simulink model "VSCMGs_trackingOrbital"  (R2019b)
settings: Solver=ode45  StartTime=0.0  StopTime=tf  FixedStep=0.01  MaxStep=0.1  RelTol=10^(-6)  EnableMultiTasking=on
InitFcn:
  | initialize
StopFcn:
  | plotting
values from neighbouring files (symbols this model uses):
  g10 = [1; 0; 0]    [initialize.m]
  g20 = [0; 1; 0]    [initialize.m]
  g30 = [0; 0; 1]    [initialize.m]
  gamma10 = 0    [initialize.m]
  gamma20 = 0    [initialize.m]
  gamma30 = 0    [initialize.m]
  h = cross(r0, v0)    [initialize.m]
  Isw = 0.1    [initialize.m]
  J = [87.252, 0, 0; 0, 85.07, 0; 0, 0, 113.565]    [initialize.m]
  K = 10^(1)*eye(3)    [initialize.m]
  mu = 10^(-20)    (= 1e-20)    [initialize.m]
  mugrav = G*(m1+m2)    (= 398583.224)    [initialize.m]
  om0 = [0; 0; 0]*(2*pi/60)    [initialize.m]
  Om0 = [500; 500; 500]*2*pi/60    [initialize.m]
  q0 = [0; 0; 0; 1]    [initialize.m]
  r0 = [8000; 0; 6000]    [initialize.m]
  s10 = [0; 1; 0]    [initialize.m]
  s20 = [1; 0; 0]    [initialize.m]
  s30 = [0; 1; 0]    [initialize.m]
  t10 = [0; 0; 1]    [initialize.m]
  t20 = [0; 0; -1]    [initialize.m]
  t30 = [-1; 0; 0]    [initialize.m]
  v0 = [0; 8.5; 0]    [initialize.m]
  Wg0 = 1    [initialize.m]
  Ws0 = 200    [initialize.m]
  Y = [0.03, 0, 0; 0, 0.13, 0; 0, 0, 0.04]    [initialize.m]
settings Model: Creator=bevilr  LastModifiedBy=bevilr
settings DataIOCC: ReturnWorkspaceOutputs=off
settings OptimizationCC: LifeSpan=inf
settings DebuggingCC: SFUnexpectedBacktrackingDiag=warning  SFNoUnconditionalDefaultTransitionDiag=warning  ArithmeticOperatorsInVariantConditions=warning
settings SFSimCC: SimUseLocalCustomCode=off  CustomCodeUndefinedFunction=UseInterfaceOnly
settings RTWCC: RTWUseLocalCustomCode=off
settings CodeAppCC: StateflowObjectComments=on
settings GRTTargetCC: TargetLangStandard=C89/C90 (ANSI)  GeneratePreprocessorConditionals=Disable all
settings ConfigComp: CovMetricSettings=dw  CovHtmlReporting=on  CovSaveCumulativeToWorkspaceVar=on  CovSaveSingleToWorkspaceVar=on  CovExternalEMLEnable=off

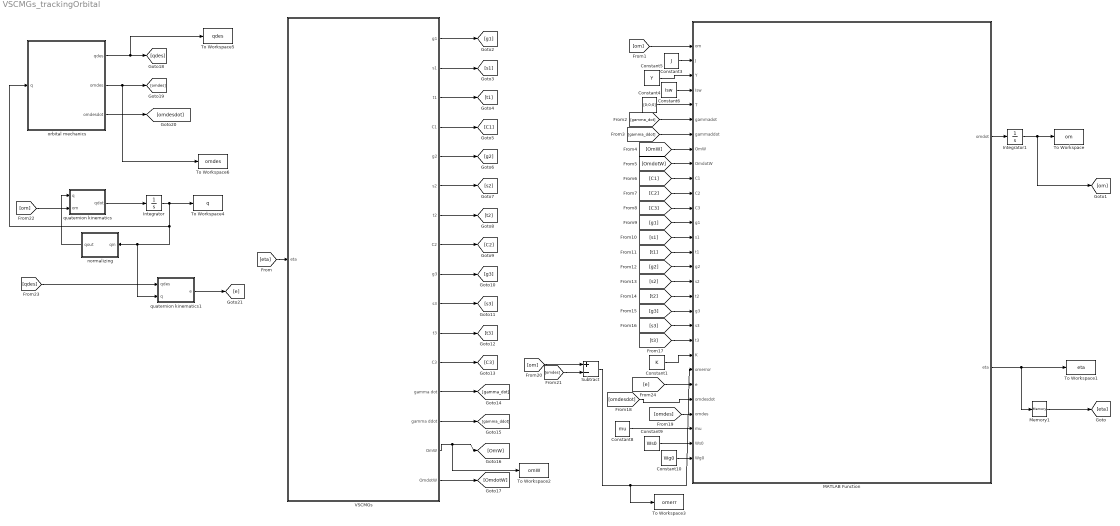
== system VSCMGs_trackingOrbital ==
  Constant1 : Constant  Value=K
  Constant10 : Constant  Value=Wg0
  Constant3 : Constant  Value=J
  Constant4 : Constant  Value=[0;0;0]
  Constant5 : Constant  Value=Y
  Constant6 : Constant  Value=Isw
  Constant8 : Constant  Value=mu
  Constant9 : Constant  Value=Ws0
  Integrator : Integrator  InitialCondition=q0
  Integrator1 : Integrator  InitialCondition=om0
  MATLAB Function : MATLAB Function  TreatAsAtomicUnit=on
  Memory1 : Memory
  Subtract : Sum  Inputs=+-
  To Workspace : ToWorkspace  VariableName=om  SampleTime=-1
  To Workspace1 : ToWorkspace  VariableName=eta  SampleTime=-1
  To Workspace2 : ToWorkspace  VariableName=omW  SampleTime=-1
  To Workspace3 : ToWorkspace  VariableName=omerr  SampleTime=-1
  To Workspace4 : ToWorkspace  VariableName=q  SampleTime=-1
  To Workspace5 : ToWorkspace  VariableName=qdes  SampleTime=-1
  To Workspace6 : ToWorkspace  VariableName=omdes  SampleTime=-1
  VSCMGs : Subsystem
  normalizing : MATLAB Function  TreatAsAtomicUnit=on
  "orbital mechanics " : Subsystem
  quaternion kinematics : MATLAB Function  TreatAsAtomicUnit=on
  quaternion kinematics1 : MATLAB Function  TreatAsAtomicUnit=on
  wires:
  Constant3/1 -> MATLAB Function/2(J)
  Constant4/1 -> MATLAB Function/5(T)
  MATLAB Function/1(omdot) -> Integrator1/1
  Constant5/1 -> MATLAB Function/3(Y)
  Constant6/1 -> MATLAB Function/4(Isw)
  Constant1/1 -> MATLAB Function/22(K)
  Integrator1/1 -> [om], To Workspace/1
  [e] -> MATLAB Function/24(e)
  MATLAB Function/2(eta) -> To Workspace1/1, Memory1/1
  Constant8/1 -> MATLAB Function/27(mu)
  Constant9/1 -> MATLAB Function/28(Ws0)
  Constant10/1 -> MATLAB Function/29(Wg0)
  Memory1/1 -> [eta]
  [om] -> MATLAB Function/1(om)
  VSCMGs/1(g1) -> [g1]
  VSCMGs/2(s1) -> [s1]
  VSCMGs/3(t1) -> [t1]
  VSCMGs/4(C1) -> [C1]
  VSCMGs/5(g2) -> [g2]
  VSCMGs/6(s2) -> [s2]
  VSCMGs/7(t2) -> [t2]
  VSCMGs/8(C2) -> [C2]
  VSCMGs/9(g3) -> [g3]
  VSCMGs/10(s3) -> [s3]
  VSCMGs/11(t3) -> [t3]
  VSCMGs/12(C3) -> [C3]
  VSCMGs/13("gamma dot ") -> [gamma_dot]
  VSCMGs/14(gamma ddot) -> [gamma_ddot]
  VSCMGs/15(OmW) -> To Workspace2/1, [OmW]
  VSCMGs/16(OmdotW) -> [OmdotW]
  [gamma_dot] -> MATLAB Function/6(gammadot)
  [gamma_ddot] -> MATLAB Function/7(gammaddot)
  [OmW] -> MATLAB Function/8(OmW)
  [OmdotW] -> MATLAB Function/9(OmdotW)
  [C1] -> MATLAB Function/10(C1)
  [C2] -> MATLAB Function/11(C2)
  [C3] -> MATLAB Function/12(C3)
  [g1] -> MATLAB Function/13(g1)
  [s1] -> MATLAB Function/14(s1)
  [t1] -> MATLAB Function/15(t1)
  [g2] -> MATLAB Function/16(g2)
  [s2] -> MATLAB Function/17(s2)
  [t2] -> MATLAB Function/18(t2)
  [g3] -> MATLAB Function/19(g3)
  [s3] -> MATLAB Function/20(s3)
  [t3] -> MATLAB Function/21(t3)
  [eta] -> VSCMGs/1(eta)
  "orbital mechanics "/1(qdes) -> To Workspace5/1, [qdes]
  "orbital mechanics "/2(omdes) -> To Workspace6/1, [omdes]
  "orbital mechanics "/3(omdesdot) -> [omdesdot]
  [omdesdot] -> MATLAB Function/25(omdesdot)
  [omdes] -> MATLAB Function/26(omdes)
  [om] -> Subtract/1
  [omdes] -> Subtract/2
  Subtract/1 -> To Workspace3/1, MATLAB Function/23(omerror)
  quaternion kinematics/1(qdot) -> Integrator/1
  [om] -> quaternion kinematics/2(om)
  Integrator/1 -> "orbital mechanics "/1(q), quaternion kinematics1/2(q), normalizing/1(qin), To Workspace4/1
  normalizing/1(qout) -> quaternion kinematics/1(q)
  quaternion kinematics1/1(e) -> [e]
  [qdes] -> quaternion kinematics1/1(qdes)

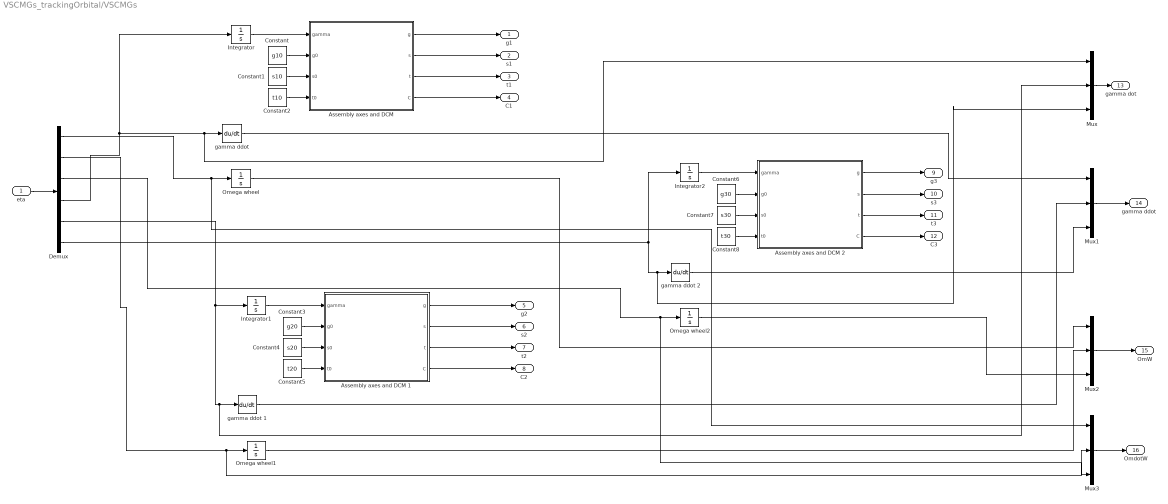
== system VSCMGs_trackingOrbital/VSCMGs ==
  eta : Inport
  "Assembly axes and DCM " : MATLAB Function  TreatAsAtomicUnit=on
  Assembly axes and DCM 1 : MATLAB Function  TreatAsAtomicUnit=on
  Assembly axes and DCM 2 : MATLAB Function  TreatAsAtomicUnit=on
  Constant : Constant  Value=g10
  Constant1 : Constant  Value=s10
  Constant2 : Constant  Value=t10
  Constant3 : Constant  Value=g20
  Constant4 : Constant  Value=s20
  Constant5 : Constant  Value=t20
  Constant6 : Constant  Value=g30
  Constant7 : Constant  Value=s30
  Constant8 : Constant  Value=t30
  Demux : Demux  Outputs=6
  Integrator : Integrator  InitialCondition=gamma10
  Integrator1 : Integrator  InitialCondition=gamma20
  Integrator2 : Integrator  InitialCondition=gamma30
  Mux{,1..3} (4 alike) : Mux  Inputs=3
  Omega wheel : Integrator  InitialCondition=Om0(1)
  Omega wheel1 : Integrator  InitialCondition=Om0(2)
  Omega wheel2 : Integrator  InitialCondition=Om0(3)
  "gamma ddot " : Derivative
  gamma ddot 1 : Derivative
  gamma ddot 2 : Derivative
  g1 : Outport  VectorParamsAs1DForOutWhenUnconnected=off
  s1 : Outport  Port=2  VectorParamsAs1DForOutWhenUnconnected=off
  t1 : Outport  Port=3  VectorParamsAs1DForOutWhenUnconnected=off
  C1 : Outport  Port=4  VectorParamsAs1DForOutWhenUnconnected=off
  g2 : Outport  Port=5  VectorParamsAs1DForOutWhenUnconnected=off
  s2 : Outport  Port=6  VectorParamsAs1DForOutWhenUnconnected=off
  t2 : Outport  Port=7  VectorParamsAs1DForOutWhenUnconnected=off
  C2 : Outport  Port=8  VectorParamsAs1DForOutWhenUnconnected=off
  g3 : Outport  Port=9  VectorParamsAs1DForOutWhenUnconnected=off
  s3 : Outport  Port=10  VectorParamsAs1DForOutWhenUnconnected=off
  t3 : Outport  Port=11  VectorParamsAs1DForOutWhenUnconnected=off
  C3 : Outport  Port=12  VectorParamsAs1DForOutWhenUnconnected=off
  "gamma dot " : Outport  Port=13  VectorParamsAs1DForOutWhenUnconnected=off
  gamma ddot : Outport  Port=14  VectorParamsAs1DForOutWhenUnconnected=off
  OmW : Outport  Port=15  VectorParamsAs1DForOutWhenUnconnected=off
  OmdotW : Outport  Port=16  VectorParamsAs1DForOutWhenUnconnected=off
  wires:
  Constant/1 -> "Assembly axes and DCM "/2(g0)
  Constant1/1 -> "Assembly axes and DCM "/3(s0)
  "Assembly axes and DCM "/3(t) -> t1/1
  Constant2/1 -> "Assembly axes and DCM "/4(t0)
  Omega wheel/1 -> Mux2/1
  Demux/1 -> Mux3/1, Omega wheel/1
  "gamma ddot "/1 -> Mux1/1
  Integrator/1 -> "Assembly axes and DCM "/1(gamma)
  "Assembly axes and DCM "/2(s) -> s1/1
  "Assembly axes and DCM "/4(C) -> C1/1
  "Assembly axes and DCM "/1(g) -> g1/1
  Demux/4 -> Mux/1, "gamma ddot "/1, Integrator/1
  Demux/5 -> Integrator1/1, Mux/2, gamma ddot 1/1
  Assembly axes and DCM 1/1(g) -> g2/1
  Assembly axes and DCM 1/4(C) -> C2/1
  Assembly axes and DCM 1/2(s) -> s2/1
  Integrator1/1 -> Assembly axes and DCM 1/1(gamma)
  gamma ddot 1/1 -> Mux1/2
  Demux/2 -> Mux3/2, Omega wheel1/1
  Omega wheel1/1 -> Mux2/2
  Constant5/1 -> Assembly axes and DCM 1/4(t0)
  Assembly axes and DCM 1/3(t) -> t2/1
  Constant4/1 -> Assembly axes and DCM 1/3(s0)
  Constant3/1 -> Assembly axes and DCM 1/2(g0)
  Demux/6 -> Integrator2/1, Mux/3, gamma ddot 2/1
  Assembly axes and DCM 2/1(g) -> g3/1
  Assembly axes and DCM 2/4(C) -> C3/1
  Assembly axes and DCM 2/2(s) -> s3/1
  Integrator2/1 -> Assembly axes and DCM 2/1(gamma)
  gamma ddot 2/1 -> Mux1/3
  Demux/3 -> Mux3/3, Omega wheel2/1
  Omega wheel2/1 -> Mux2/3
  Constant8/1 -> Assembly axes and DCM 2/4(t0)
  Assembly axes and DCM 2/3(t) -> t3/1
  Constant7/1 -> Assembly axes and DCM 2/3(s0)
  Constant6/1 -> Assembly axes and DCM 2/2(g0)
  Mux/1 -> "gamma dot "/1
  Mux1/1 -> gamma ddot/1
  Mux2/1 -> OmW/1
  Mux3/1 -> OmdotW/1
  eta/1 -> Demux/1

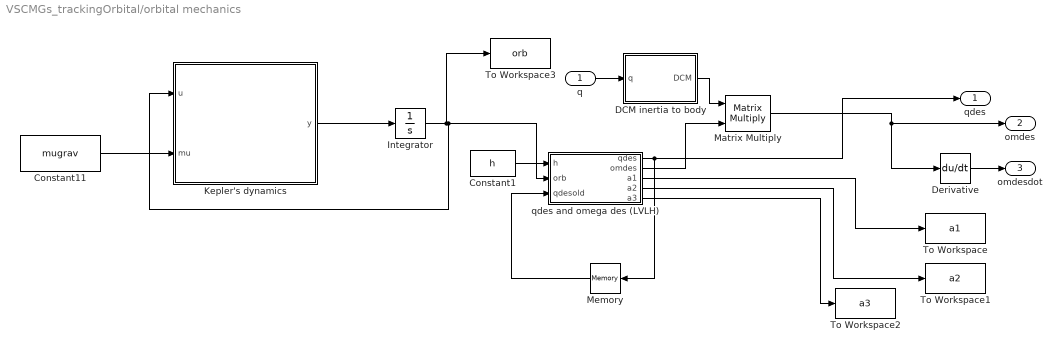
== system VSCMGs_trackingOrbital/orbital mechanics  ==
  q : Inport
  Constant1 : Constant  Value=h
  Constant11 : Constant  Value=mugrav
  DCM inertia to body : MATLAB Function  TreatAsAtomicUnit=on
  Derivative : Derivative
  Integrator : Integrator  InitialCondition=[r0; v0]
  Kepler's dynamics : MATLAB Function  TreatAsAtomicUnit=on
  Matrix Multiply : Product  Multiplication=Matrix(*)
  Memory : Memory  InitialCondition=[0;0;0;1]
  To Workspace : ToWorkspace  VariableName=a1  SampleTime=-1
  To Workspace1 : ToWorkspace  VariableName=a2  SampleTime=-1
  To Workspace2 : ToWorkspace  VariableName=a3  SampleTime=-1
  To Workspace3 : ToWorkspace  VariableName=orb  SampleTime=-1
  "qdes and omega des (LVLH) " : MATLAB Function  TreatAsAtomicUnit=on
  qdes : Outport  VectorParamsAs1DForOutWhenUnconnected=off
  omdes : Outport  Port=2  VectorParamsAs1DForOutWhenUnconnected=off
  omdesdot : Outport  Port=3  VectorParamsAs1DForOutWhenUnconnected=off
  wires:
  Kepler's dynamics/1(y) -> Integrator/1
  Integrator/1 -> To Workspace3/1, Kepler's dynamics/1(u), "qdes and omega des (LVLH) "/2(orb)
  Constant11/1 -> Kepler's dynamics/2(mu)
  Constant1/1 -> "qdes and omega des (LVLH) "/1(h)
  "qdes and omega des (LVLH) "/1(qdes) -> Memory/1, qdes/1
  Derivative/1 -> omdesdot/1
  "qdes and omega des (LVLH) "/3(a1) -> To Workspace/1
  "qdes and omega des (LVLH) "/4(a2) -> To Workspace1/1
  "qdes and omega des (LVLH) "/5(a3) -> To Workspace2/1
  Memory/1 -> "qdes and omega des (LVLH) "/3(qdesold)
  q/1 -> DCM inertia to body/1(q)
  "qdes and omega des (LVLH) "/2(omdes) -> Matrix Multiply/2
  Matrix Multiply/1 -> omdes/1, Derivative/1
  DCM inertia to body/1(DCM) -> Matrix Multiply/1

== matlab function VSCMGs_trackingOrbital/MATLAB Function ==
  data: om input; J input; Y input; Isw input; omdot output; T input; gammadot input size=3; gammaddot input size=3; OmW input size=3; OmdotW input size=3; C1 input size=[3,3]; C2 input size=[3,3]; C3 input size=[3,3]; g1 input size=3; s1 input size=3; t1 input size=3; g2 input size=3; s2 input size=3; t2 input size=3; g3 input size=3; s3 input size=3; t3 input size=3; K input; omerror input; e input; omdesdot input; eta output; omdes input; mu input; Ws0 input; Wg0 input
function [omdot, eta] = fulldynamics(om, J, Y, Isw, T, gammadot, gammaddot, OmW, OmdotW, ...
                     C1, C2, C3, g1, s1, t1, g2, s2, t2, g3, s3, t3, K, omerror, e, omdesdot, omdes, mu, Ws0, Wg0)

eta = [0; 0; 0; 0; 0; 0];

%omdot = inv(J)*(-cross(om, J*om)+T);
omdot = inv(J+C1*Y*C1'+C2*Y*C2'+C3*Y*C3')*(-Y(1,1)*gammaddot(1)*g1-Y(1,1)*gammaddot(2)*g2-Y(1,1)*gammaddot(3)*g3 ...
                                           -Isw*OmdotW(1)*s1-Isw*OmdotW(2)*s2-Isw*OmdotW(3)*s3 ...
                                           -Isw*OmW(1)*gammadot(1)*t1-Isw*OmW(2)*gammadot(2)*t2-Isw*OmW(3)*gammadot(3)*t3 ...
                                           -(Y(2,2)-Y(3,3))*gammadot(1)*(t1*s1'+s1*t1')*om ...
                                           -(Y(2,2)-Y(3,3))*gammadot(2)*(t2*s2'+s2*t2')*om ...
                                           -(Y(2,2)-Y(3,3))*gammadot(3)*(t3*s3'+s3*t3')*om ...
                                           -cross(om, (J+C1*Y*C1'+C2*Y*C2'+C3*Y*C3')*om) ...
                                           -Y(1,1)*gammadot(1)*cross(om, g1)-Y(1,1)*gammadot(2)*cross(om, g2)-Y(1,1)*gammadot(3)*cross(om, g3) ...
                                           -Isw*OmW(1)*cross(om, s1)-Isw*OmW(2)*cross(om, s2)-Isw*OmW(3)*cross(om, s3) + T);
 
B = [g1, g2, g3]*diag([Y(1,1);Y(1,1);Y(1,1)]);                                       

C = [t1, t2, t3]*diag([Isw;Isw;Isw])*diag([OmW(1);OmW(2);OmW(3)]) + [0, -om(3), om(2); om(3), 0, -om(1); -om(2), om(1), 0]*...
    [g1, g2, g3]*diag([Y(1,1);Y(1,1);Y(1,1)]) + (1/2)*[(t1*s1'+s1*t1')*(om+omdes), (t2*s2'+s2*t2')*(om+omdes), (t3*s3'+s3*t3')*(om+omdes)]*...
    (diag([Y(2,2);Y(2,2);Y(2,2)]) - diag([Y(3,3);Y(3,3);Y(3,3)]));

D = [s1, s2, s3]*diag([Isw;Isw;Isw]);

Q = [D, C];
                                       
Tmed = T + K*omerror + e - cross(om,  ((J+C1*Y*C1'+C2*Y*C2'+C3*Y*C3')*om + Isw*OmW(1)*s1 + Isw*OmW(2)*s2 + + Isw*OmW(3)*s3)) + ...
        - (J+C1*Y*C1'+C2*Y*C2'+C3*Y*C3')*omdesdot ;%- B*[gammaddot(1); gammaddot(2); gammaddot(3)]; (not needed, as discussed)
 

%singularity indicator
delta = det(C*C');

%weight matrix
W = [Ws0*exp(-mu*delta) 0 0 0 0 0; 0 Ws0*exp(-mu*delta) 0 0 0 0; 0 0 Ws0*exp(-mu*delta) 0 0 0; ...
    0 0 0 Wg0 0 0; 0 0 0 0 Wg0 0; 0 0 0 0 0 Wg0];

%control variable (wheels' accelerations and gimbal rates)
eta = W*Q'*inv(Q*W*Q')*Tmed;

== matlab function VSCMGs_trackingOrbital/VSCMGs/Assembly axes and DCM  ==
  data: gamma input; g output; s output; t output; C output; g0 input; s0 input; t0 input
function [g, s, t, C] = fcn(gamma, g0, s0, t0)
%#codegen

g = g0;
s = cos(gamma)*s0 + sin(gamma)*t0;
t = cos(gamma)*t0 - sin(gamma)*s0;
C = [g, s, t];

== matlab function VSCMGs_trackingOrbital/VSCMGs/Assembly axes and DCM 2 ==
  data: gamma input; g output; s output; t output; C output; g0 input; s0 input; t0 input
function [g, s, t, C] = fcn(gamma, g0, s0, t0)
%#codegen

g = g0;
s = cos(gamma)*s0 + sin(gamma)*t0;
t = cos(gamma)*t0 - sin(gamma)*s0;
C = [g, s, t];

== matlab function VSCMGs_trackingOrbital/orbital mechanics /Kepler's dynamics ==
  data: u input; y output; mu input
function y = kepler(u, mu)
%#codegen

r = u(1:3);

y = [u(4:6);-mu*r/norm(r)^3];

== matlab function VSCMGs_trackingOrbital/VSCMGs/Assembly axes and DCM 1 ==
  data: gamma input; g output; s output; t output; C output; g0 input; s0 input; t0 input
function [g, s, t, C] = fcn(gamma, g0, s0, t0)
%#codegen

g = g0;
s = cos(gamma)*s0 + sin(gamma)*t0;
t = cos(gamma)*t0 - sin(gamma)*s0;
C = [g, s, t];

== matlab function VSCMGs_trackingOrbital/orbital mechanics /qdes and omega des (LVLH)  ==
  data: h input; qdes output; orb input; omdes output; a1 output; a2 output; a3 output; qdesold input
function [qdes, omdes, a1, a2, a3] = fcn(h, orb, qdesold)

q = [1; 0; 0; 0];
qdes = [1; 0; 0; 0];

a3 = -orb(1:3)/norm(orb(1:3));
a2 = -h/norm(h);
a1 = cross(a2, a3);

%direction cosine matrix between LVLH and ECI
dcm = [a1, a2, a3]';

%%%%%%%%%%%%%%%%%%%%%%%%%%%%%%%%%%%%%%%%%%%%%%%%%%%%%%%
%transforming into quaternion (modified Matlab function)
q(4) =  0; 

tr = trace(dcm);

if (tr > 0)
    sqtrp1 = sqrt( tr + 1.0 );

    q(1) = 0.5*sqtrp1; 
    q(2) = (dcm(2, 3) - dcm(3, 2))/(2.0*sqtrp1);
    q(3) = (dcm(3, 1) - dcm(1, 3))/(2.0*sqtrp1); 
    q(4) = (dcm(1, 2) - dcm(2, 1))/(2.0*sqtrp1); 
else
    d = diag(dcm);
    if ((d(2) > d(1)) && (d(2) > d(3)))
        % max value at dcm(2,2,i)
        sqdip1 = sqrt(d(2) - d(1) - d(3) + 1.0 );

        q(3) = 0.5*sqdip1; 

        if ( sqdip1 ~= 0 )
            sqdip1 = 0.5/sqdip1;
        end

        q(1) = (dcm(3, 1) - dcm(1, 3))*sqdip1; 
        q(2) = (dcm(1, 2) + dcm(2, 1))*sqdip1; 
        q(4) = (dcm(2, 3) + dcm(3, 2))*sqdip1; 
    elseif (d(3) > d(1))
        % max value at dcm(3,3,i)
        sqdip1 = sqrt(d(3) - d(1) - d(2) + 1.0 );

        q(4) = 0.5*sqdip1; 

        if ( sqdip1 ~= 0 )
            sqdip1 = 0.5/sqdip1;
        end

        q(1) = (dcm(1, 2) - dcm(2, 1))*sqdip1;
        q(2) = (dcm(3, 1) + dcm(1, 3))*sqdip1; 
        q(3) = (dcm(2, 3) + dcm(3, 2))*sqdip1; 
    else
        % max value at dcm(1,1,i)
        sqdip1 = sqrt(d(1) - d(2) - d(3) + 1.0 );

        q(2) = 0.5*sqdip1; 

        if ( sqdip1 ~= 0 )
            sqdip1 = 0.5/sqdip1;
        end

        q(1) = (dcm(2, 3) - dcm(3, 2))*sqdip1; 
        q(3) = (dcm(1, 2) + dcm(2, 1))*sqdip1; 
        q(4) = (dcm(3, 1) + dcm(1, 3))*sqdip1; 
    end
end
%%%%%%%%%MODIFIED FROM MATLAB
%%%%%%%%%%%%%%%%%%%%%%%%%%%%%%%%%%%%%%%%%%%%%%%%%%%%%%%

%reordering to match our definition of quaternion
qdes = [q(2); q(3); q(4); q(1)];

if dot(qdesold, qdes) < 0
    qdes = -qdes;
end

%angular velocity of LVLH in inertial
omdes = (norm(h)/norm(orb(1:3))^2)*(-a2);

== matlab function VSCMGs_trackingOrbital/quaternion kinematics ==
  data: q input; qdot output; om input
function qdot = fcn(q, om)
%#codegen

qdot = (1/2)*[q(4) -q(3) q(2) q(1);...
              q(3) q(4) -q(1) q(2);...
              -q(2) q(1) q(4) q(3);
              -q(1) -q(2) -q(3) q(4)]*[om; 0];

== matlab function VSCMGs_trackingOrbital/normalizing ==
  data: qin input; qout output
function qout = fcn(qin)
%#codegen

qout = qin/norm(qin);

== matlab function VSCMGs_trackingOrbital/quaternion kinematics1 ==
  data: qdes input; q input; e output
function e = fcn(qdes, q)
%#codegen

e = [qdes(4) -qdes(3) qdes(2);...
     qdes(3) qdes(4) -qdes(1);...
     -qdes(2) qdes(1) qdes(4);
     -qdes(1) -qdes(2) -qdes(3)]'*q;

== matlab function VSCMGs_trackingOrbital/orbital mechanics /DCM inertia to body ==
  data: q input; DCM output
function DCM = Inertia2Body(q)

DCM = [1-2*(q(2)^2+q(3)^2) 2*(q(1)*q(2)+q(3)*q(4)) 2*(q(1)*q(3)-q(2)*q(4));
     2*(q(1)*q(2)-q(3)*q(4)) 1-2*(q(1)^2+q(3)^2) 2*(q(2)*q(3)+q(1)*q(4));
     2*(q(1)*q(3)+q(2)*q(4))  2*(q(2)*q(3)-q(1)*q(4)) 1-2*(q(1)^2+q(2)^2)]';
